simulink model "tester"  (Simulink 7.3)
settings: Solver=ode1  SolverMode=SingleTasking  StartTime=0.0  StopTime=4  FixedStep=0.001  RelTol=1e-3
values from neighbouring files (symbols this model uses):
  Beq = 0.0015*6    (= 0.009)    [Sve ikad.m]    (also in matlab.mat = 0.0075)
  Eff_G = 0.9    [Sve ikad.m]    (also in matlab.mat)
  Eff_M = 0.69    [Sve ikad.m]    (also in matlab.mat)
  Jeq = 2e-3    (= 0.002)    [Sve ikad.m]    (also in matlab.mat)
  Ke = 0.0076776    [Sve ikad.m]    (also in matlab.mat)
  Kg = 70    [Sve ikad.m]    (also in matlab.mat)
  Km = 0.007683    [Sve ikad.m]    (also in matlab.mat)
  Ra = 2.6    [Sve ikad.m]    (also in matlab.mat)
undefined symbols (not defined in the file or in its folder): MultiQ, PCI, Quanser
libraries: rtwinlib x2
settings Model: Creator=Labos  LastModifiedBy=Mehatronicki Sustavi  SimulationMode=external  ExtModeTrigDuration=1000000
settings HardwareCC: ProdIntDivRoundTo=Zero  ProdEndianess=LittleEndian  ProdHWDeviceType=Generic->32-bit x86 compatible
settings RTWCC: SystemTargetFile=rtwin.tlc  TemplateMakefile=rtwin.tmf  Description=Real-Time Windows Target  ProcessScript=rtwin_make_rtw_hook  RTWCompilerOptimization=On
settings CodeAppCC: MaxIdLength=95
settings RTWinTargetCC: TargetFunctionLibrary=ANSI_C  PortableWordSizes=off

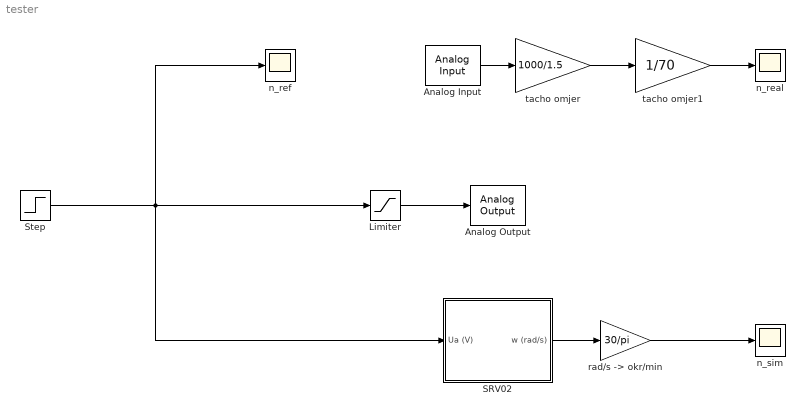
== system tester ==
  Analog Input : rtwinlib/Analog Input  SampleTime=0.001  DrvName=Quanser/MultiQ-PCI  DrvAddress=4294967295  DrvOptions=zeros(1,0)  Channels=4  RangeMode=1  VoltRange=1  DataType=1
      settings: AttributesFormatString=Quanser\nMultiQ-PCI [auto]
  Analog Output : rtwinlib/Analog Output  SampleTime=0.001  DrvName=Quanser/MultiQ-PCI  DrvAddress=4294967295  DrvOptions=zeros(1,0)  Channels=1  RangeMode=1  VoltRange=1  InitialValue=0  FinalValue=0
      settings: AttributesFormatString=Quanser\nMultiQ-PCI [auto]
  Limiter : Saturate  UpperLimit=6  LowerLimit=-6
  "SRV02 " : Subsystem
  Step : Step  After=4
  n_real : Scope
      settings: TimeRange=5  YMin=0  YMax=30  SaveName=n_real_test  DataFormat=Array  SampleInput=on
  n_ref : Scope
      settings: TimeRange=5  YMin=0  YMax=30  SaveName=n_ref  DataFormat=Array  SampleInput=on
  n_sim : Scope
      settings: TimeRange=5  YMin=0  YMax=30  SaveName=n_sim_test  DataFormat=Array  SampleInput=on
  "rad/s -> okr/min" : Gain  Gain=30/pi
  tacho omjer : Gain  Gain=1000/1.5
  tacho omjer1 : Gain  Gain=1/70
  wires:
  Limiter/1 -> Analog Output/1
  Step/1 -> Limiter/1, n_ref/1, "SRV02 "/1(Ua (V))
  "SRV02 "/1(w (rad/s)) -> "rad/s -> okr/min"/1
  "rad/s -> okr/min"/1 -> n_sim/1
  Analog Input/1 -> tacho omjer/1
  tacho omjer/1 -> tacho omjer1/1
  tacho omjer1/1 -> n_real/1

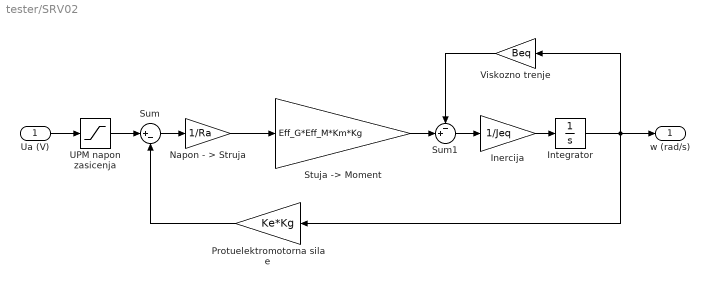
== system tester/SRV02  ==
  Ua (V) : Inport
  Inercija : Gain  Gain=1/Jeq
  Integrator : Integrator
  Napon - > Struja : Gain  Gain=1/Ra
  Protuelektromotorna sila e : Gain  Gain=Ke*Kg
  "Stuja -> Moment" : Gain  Gain=Eff_G*Eff_M*Km*Kg
  Sum : Sum  Inputs=|+-
  Sum1 : Sum  Inputs=-+|
  UPM napon zasicenja : Saturate  UpperLimit=6  LowerLimit=-6
  Viskozno trenje : Gain  Gain=Beq
  w (rad/s) : Outport
  wires:
  Sum1/1 -> Inercija/1
  "Stuja -> Moment"/1 -> Sum1/2
  Inercija/1 -> Integrator/1
  UPM napon zasicenja/1 -> Sum/1
  Napon - > Struja/1 -> "Stuja -> Moment"/1
  Ua (V)/1 -> UPM napon zasicenja/1
  Sum/1 -> Napon - > Struja/1
  Viskozno trenje/1 -> Sum1/1
  Protuelektromotorna sila e/1 -> Sum/2
  Integrator/1 -> w (rad/s)/1, Protuelektromotorna sila e/1, Viskozno trenje/1
